simulink model "stateSpace1"  (R2020a)
settings: Solver=VariableStepAuto  StartTime=0.0  StopTime=10  RelTol=1e-3  EnableMultiTasking=on
values from neighbouring files (symbols this model uses):
  g = 9.80665    [modelParameters.m]
  I_r_A = I_r_B + m_r*l_AB^2    (= 0.00169018666667)    [modelParameters.m]
  I_w_A = I_w_C + m_w*l_AC^2    (= 0.001261425)    [modelParameters.m]
  I_w_C = 0.5*m_w*R^2    (= 8.6875e-05)    [modelParameters.m]
  l_AB = l/2    (= 0.065)    [modelParameters.m]
  l_AC = l    (= 0.13)    [modelParameters.m]
  m_r = 0.2948    [modelParameters.m]
  m_w = 0.0695    [modelParameters.m]
settings Model: Creator=bkhusain  LastModifiedBy=mmarathe
settings DataIOCC: LimitDataPoints=on  MaxDataPoints=10000
settings OptimizationCC: LifeSpan=inf
settings DebuggingCC: AllowSymbolicDim=off  SFUnexpectedBacktrackingDiag=warning  SFNoUnconditionalDefaultTransitionDiag=warning  SFExecutionAtInitializationDiag=none  ArithmeticOperatorsInVariantConditions=warning
settings SFSimCC: SimUseLocalCustomCode=off  CustomCodeUndefinedFunction=UseInterfaceOnly
settings RTWCC: RTWUseLocalCustomCode=off
settings CodeAppCC: StateflowObjectComments=on
settings GRTTargetCC: TargetLangStandard=C89/C90 (ANSI)
settings ConfigComp: CovMetricSettings=dw  CovHtmlReporting=on  CovSaveCumulativeToWorkspaceVar=on  CovSaveSingleToWorkspaceVar=on  CovExternalEMLEnable=off  CovSFcnEnable=off
settings SimscapeCC: SimscapeLogType=all  SimscapeLogSimulationStatistics=on  SimscapeLogDataHistory=10000

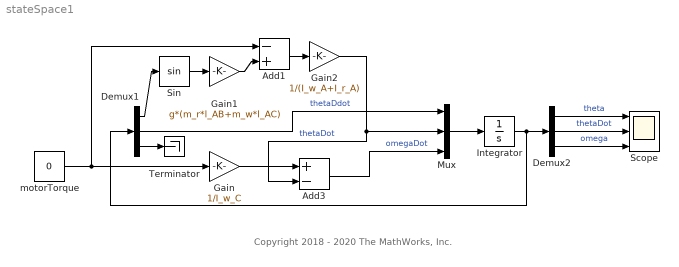
== system stateSpace1 ==
  note: Copyright 2018 - 2020 The MathWorks, Inc.
  Add1 : Sum  Inputs=-+
  Add3 : Sum  Inputs=+-
  Demux1 : Demux  Outputs=3
  Demux2 : Demux  Outputs=3
  Gain : Gain  Gain=1/I_w_C
  Gain1 : Gain  Gain=g*(m_r*l_AB+m_w*l_AC)
  Gain2 : Gain  Gain=1/(I_w_A+I_r_A)
  Integrator : Integrator  InitialCondition=[10*pi/180; 0; 0]
  Mux : Mux  Inputs=3
  Scope : Scope  NumInputPorts=3
  Sin : Trigonometry  OutputSignalType=real
  Terminator : Terminator
  motorTorque : Constant  Value=0
  wires:
  Demux2/1 -> Scope/1  "theta"
  Demux2/3 -> Scope/3  "omega"
  Integrator/1 -> Demux2/1, Demux1/1
  Demux2/2 -> Scope/2  "thetaDot"
  motorTorque/1 -> Add1/1, Gain/1
  Gain2/1 -> Add3/2, Mux/2  "thetaDot"
  Mux/1 -> Integrator/1
  Demux1/2 -> Mux/1  "thetaDdot"
  Add3/1 -> Mux/3  "omegaDot"
  Demux1/1 -> Sin/1
  Gain1/1 -> Add1/2
  Gain/1 -> Add3/1
  Add1/1 -> Gain2/1
  Sin/1 -> Gain1/1
  Demux1/3 -> Terminator/1
